simulink model "Triple_rotor_Tilerotor_model"  (R2024b)
settings: Solver=ode45  StartTime=0.0  StopTime=100  FixedStep=1e-3  RelTol=1e-3
values from neighbouring files (symbols this model uses):
  para =     [Triple_Rotors_Tilrotor_Parameters.mat]
undefined symbols (not defined in the file or in its folder): initial_height, initial_pitch, initial_vx, magnitude, rot2
libraries: simulink x9, slpidlib x5, matrix_library x4, vrlib x1
(part 2 of 3)

== system Triple_rotor_Tilerotor_model/attack_down ==
  note: 不要使用阶跃输入，会变得不幸
  Bus Creator : BusCreator  Inputs=4
  Constant : Constant  Value=Aerodynamic_switch
  Constant1 : Constant  Value=initial_theta
  Constant2 : Constant  Value=1000
  Constant3 : Constant  Value=0
  Constant4 : Constant  Value=100
  Gain : Gain  Gain=pi/180
  Gain1 : Gain  Gain=pi/180
  Ramp : simulink/Sources/Ramp  slope=slope  start=0  InitialOutput=initial_theta
  Saturation2 : Saturate  UpperLimit=inf  LowerLimit=0
  Step : Step  Commented=on  Time=0  Before=initial_theta  After=0  SampleTime=0
  Vx* : Constant  Value=100
  gamma* : Constant  Value=0
  height : Constant  Value=1000
  tag scope: Aerodynamic_switch=global, command=global, initial_Vx=global, initial_gamma=global, initial_height=global, initial_theta=global
  wires:
  Saturation2/1 -> Bus Creator/4  "theta*"
  height/1 -> Bus Creator/2  "height*"
  gamma*/1 -> Bus Creator/3  "gamma*"
  Vx*/1 -> Bus Creator/1  "Vx*"
  Bus Creator/1 -> [command]
  Constant/1 -> [Aerodynamic_switch]
  Constant1/1 -> Gain1/1
  Constant3/1 -> Gain/1
  Constant2/1 -> [initial_height]
  Constant4/1 -> [initial_Vx]
  Gain/1 -> [initial_gamma]
  Gain1/1 -> [initial_theta]
  Ramp/1 -> Saturation2/1

== system Triple_rotor_Tilerotor_model/attack_up ==
  Bus Creator : BusCreator  Inputs=4
  Constant : Constant  Value=Aerodynamic_switch
  Constant1 : Constant  Value=0
  Constant2 : Constant  Value=1000
  Constant3 : Constant  Value=0
  Constant4 : Constant  Value=100
  Step : Step  Time=0  After=final_theta  SampleTime=0
  Vx* : Constant  Value=100
  gamma* : Constant  Value=0
  height : Constant  Value=1000
  tag scope: Aerodynamic_switch=global, command=global, initial_Vx=global, initial_gamma=global, initial_height=global, initial_theta=global
  wires:
  Step/1 -> Bus Creator/4  "theta*"
  height/1 -> Bus Creator/2  "height*"
  gamma*/1 -> Bus Creator/3  "gamma*"
  Vx*/1 -> Bus Creator/1  "Vx*"
  Bus Creator/1 -> [command]
  Constant/1 -> [Aerodynamic_switch]
  Constant1/1 -> [initial_theta]
  Constant3/1 -> [initial_gamma]
  Constant2/1 -> [initial_height]
  Constant4/1 -> [initial_Vx]

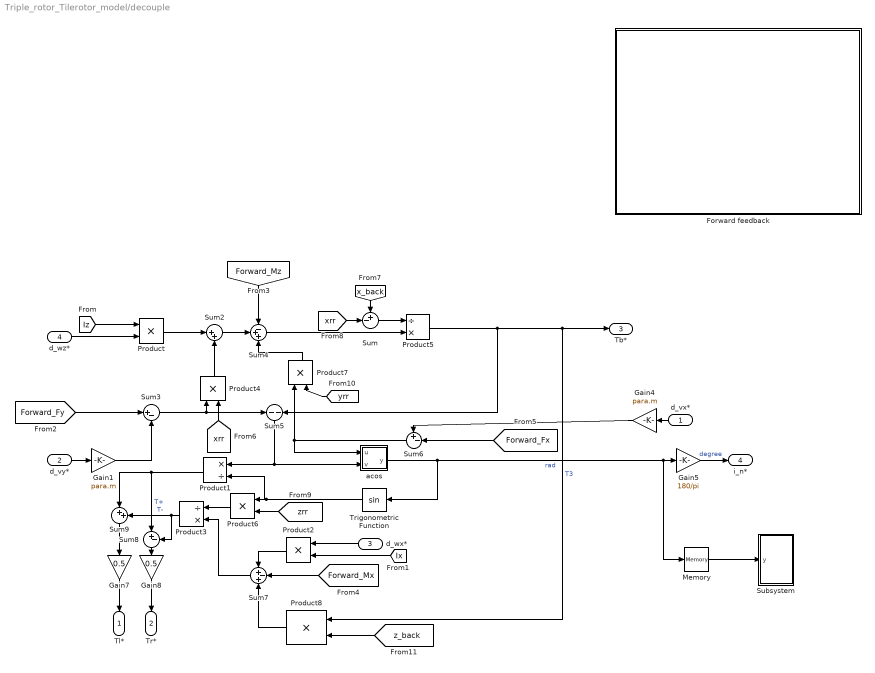
== system Triple_rotor_Tilerotor_model/decouple ==
  d_vx* : Inport
  d_vy* : Inport  Port=2
  d_wx* : Inport  Port=3
  d_wz* : Inport  Port=4
  Forward feedback : Subsystem
  Gain1 : Gain  Gain=para.m
  Gain4 : Gain  Gain=para.m
  Gain5 : Gain  Gain=180/pi
  Gain7 : Gain  Gain=0.5
  Gain8 : Gain  Gain=0.5
  Memory : Memory  InitialCondition=initial_i_n
  Product{,2,4,6..8} (6 alike) : Product
  Product1 : Product  Inputs=*/
  Product3 : Product  Inputs=/*
  Product5 : Product  Inputs=/*
  Subsystem : Subsystem
  Sum : Sum  Inputs=+-|
  Sum2 : Sum  Inputs=|++
  Sum3 : Sum  Inputs=|+-
  Sum4 : Sum  Inputs=-++
  Sum5 : Sum  Inputs=-|-
  Sum6 : Sum  Inputs=+-|
  Sum7 : Sum  Inputs=+-+
  Sum8 : Sum  Inputs=|+-
  Sum9 : Sum  Inputs=|++
  Trigonometric Function : Trigonometry
  acos : MATLAB Function  TreatAsAtomicUnit=on
  Tl* : Outport
  Tr* : Outport  Port=2
  Tb* : Outport  Port=3
  i_n* : Outport  Port=4
  wires:
  Product1/1 -> Sum8/1, Sum9/1  "T+"
  Product/1 -> Sum2/1
  [Forward_Mx] -> Sum7/2
  Gain4/1 -> Sum6/1
  Product3/1 -> Sum9/2, Sum8/2  "T-"
  [Iz] -> Product/1
  Gain1/1 -> Sum3/2
  Gain8/1 -> Tr*/1
  [Forward_Fx] -> Sum6/2
  Sum4/1 -> Product5/2
  Gain5/1 -> i_n*/1  "degree"
  [Ix] -> Product2/2
  d_vy*/1 -> Gain1/1
  Sum7/1 -> Product3/2
  d_vx*/1 -> Gain4/1
  Sum8/1 -> Gain8/1
  Sum3/1 -> Sum5/1, Product4/1
  Gain7/1 -> Tl*/1
  Product2/1 -> Sum7/1
  Trigonometric Function/1 -> Product1/2, Product6/1
  Product6/1 -> Product3/1
  d_wx*/1 -> Product2/1
  Sum9/1 -> Gain7/1
  Product4/1 -> Sum2/2
  [xrr] -> Product4/2
  [x_back] -> Sum/1
  [xrr] -> Sum/2
  Sum/1 -> Product5/1
  [zrr] -> Product6/2
  d_wz*/1 -> Product/2
  [yrr] -> Product7/2
  Product7/1 -> Sum4/3
  [z_back] -> Product8/2
  Product8/1 -> Sum7/3
  Product5/1 -> Sum5/2, Tb*/1, Product8/1  "T3"
  acos/1(y) -> Trigonometric Function/1, Memory/1, Gain5/1  "rad"
  Memory/1 -> Subsystem/1(y)
  Sum5/1 -> acos/2(v), Product1/1
  Sum6/1 -> acos/1(u), Product7/1
  [Forward_Mz] -> Sum4/1
  Sum2/1 -> Sum4/2
  [Forward_Fy] -> Sum3/1

== system Triple_rotor_Tilerotor_model/elevate2 ==
  Bus Creator : BusCreator  Inputs=4
  Constant : Constant  Value=Aerodynamic_switch
  Constant1 : Constant  Value=4
  Constant2 : Constant  Value=1000
  Constant3 : Constant  Value=0
  Constant4 : Constant  Value=100
  Constant5 : Constant  Value=-40
  Continuous Pulse Generator : DiscretePulseGenerator  PulseType=Time based  Amplitude=max_gamma  Period=200  PulseWidth=2  PhaseDelay=20
  Gain : Gain  Gain=pi/180
  Gain1 : Gain  Gain=pi/180
  Vx* : Constant  Value=100
  height : Constant  Value=1000
  theta*1 : Constant  Value=4
  tag scope: Aerodynamic_switch=global, command=global, in=global, initial_Vx=global, initial_gamma=global, initial_height=global, initial_theta=global
  wires:
  theta*1/1 -> Bus Creator/4  "theta*"
  height/1 -> Bus Creator/2  "height*"
  Continuous Pulse Generator/1 -> Bus Creator/3  "gamma*"
  Vx*/1 -> Bus Creator/1  "Vx*"
  Bus Creator/1 -> [command]
  Constant/1 -> [Aerodynamic_switch]
  Constant1/1 -> Gain1/1
  Constant3/1 -> Gain/1
  Constant2/1 -> [initial_height]
  Constant4/1 -> [initial_Vx]
  Gain/1 -> [initial_gamma]
  Gain1/1 -> [initial_theta]
  Constant5/1 -> [in]

== system Triple_rotor_Tilerotor_model/height ==
  Bus Creator : BusCreator  Inputs=4
  Constant : Constant  Value=Aerodynamic_switch
  Constant2 : Constant  Value=1000
  Constant4 : Constant  Value=100
  Constant5 : Constant  Value=0
  Constant6 : Constant  Value=0
  Gain : Gain  Gain=pi/180
  Gain1 : Gain  Gain=pi/180
  Ramp : simulink/Sources/Ramp  slope=slope  start=0  InitialOutput=1000
  Saturation2 : Saturate  UpperLimit=final_y  LowerLimit=0
  dx* : Constant  Value=100
  gamma* : Constant  Value=0
  theta* : Constant  Value=4
  tag scope: Aerodynamic_switch=global, command=global, initial_Vx=global, initial_gamma=global, initial_height=global, initial_theta=global
  wires:
  theta*/1 -> Bus Creator/4  "theta*"
  Saturation2/1 -> Bus Creator/2  "height*"
  gamma*/1 -> Bus Creator/3  "gamma*"
  Ramp/1 -> Saturation2/1
  dx*/1 -> Bus Creator/1  "Vx*"
  Bus Creator/1 -> [command]
  Constant/1 -> [Aerodynamic_switch]
  Constant2/1 -> [initial_height]
  Constant4/1 -> [initial_Vx]
  Gain1/1 -> [initial_theta]
  Constant5/1 -> Gain1/1
  Constant6/1 -> Gain/1
  Gain/1 -> [initial_gamma]

== system Triple_rotor_Tilerotor_model/observe ==
  In1 : Inport
  In2 : Inport  Port=2
  Bus Creator{1..7} (7 alike) : BusCreator  Inputs=2
  Bus Selector : BusSelector  OutputSignals=vx,vy,vz,gamma,psi,theta,wx,wy,wz
  Bus Selector1 : BusSelector  OutputSignals=vx_d,vy_d,gamma_d,theta_d
  Bus Selector2 : BusSelector  OutputSignals=wx_d,wz_d
  Demux2 : Demux  Outputs=2
  Gain5 : Gain  Gain=180/pi
  Gain6 : Gain  Gain=180/pi
  Gain7 : Gain  Gain=180/pi
  Matrix Multiply : Product  Multiplication=Matrix(*)
  Sum : Sum  Inputs=|++
  rot2(pitch) : MATLABFcn  MATLABFcn=rot2(u)  OutputDimensions=[2 2]  Output1D=off
  vx : Outport
  vy : Outport  Port=2
  <vz> : Outport  Port=3
  gamma : Outport  Port=4
  psi : Outport  Port=5
  theta : Outport  Port=6
  wx : Outport  Port=7
  <wy> : Outport  Port=8
  wz : Outport  Port=9
  i_n : Outport  Port=10
  wires:
  Bus Selector/5 -> Gain7/1  "<psi>"
  Bus Selector2/2 -> Bus Creator6/2  "<wz_d>"
  Bus Selector/7 -> Bus Creator5/1  "<wx>"
  Bus Selector/2 -> Bus Creator7/2  "<vy>"
  Bus Creator4/1 -> Gain6/1
  Bus Selector/9 -> Bus Creator6/1  "<wz>"
  Bus Creator3/1 -> Gain5/1
  Bus Selector/4 -> Bus Creator3/1  "<gamma>"
  Bus Selector1/1 -> Bus Creator1/2  "<vx_d>"
  Bus Selector/6 -> rot2(pitch)/1, Bus Creator4/1  "<theta>"
  Bus Creator7/1 -> Matrix Multiply/2
  rot2(pitch)/1 -> Matrix Multiply/1
  Demux2/2 -> Bus Creator2/1
  Gain6/1 -> theta/1  "theta"
  Bus Creator6/1 -> wz/1  "wz"
  [desire2] -> Bus Selector2/1
  Bus Selector/3 -> <vz>/1  "<vz>"
  Bus Selector1/3 -> Bus Creator3/2  "<gamma_d>"
  Bus Selector1/4 -> Bus Creator4/2  "<theta_d>"
  Bus Creator2/1 -> vy/1  "vy"
  Matrix Multiply/1 -> Demux2/1
  Bus Selector2/1 -> Bus Creator5/2  "<wx_d>"
  Demux2/1 -> Bus Creator1/1
  Bus Creator5/1 -> wx/1  "wx"
  Bus Selector1/2 -> Bus Creator2/2  "<vy_d>"
  [desire] -> Bus Selector1/1
  Bus Selector/8 -> <wy>/1  "<wy>"
  Bus Selector/1 -> Bus Creator7/1  "<vx>"
  In1/1 -> Bus Selector/1
  Gain7/1 -> psi/1  "psi"
  Gain5/1 -> gamma/1  "gamma"
  Bus Creator1/1 -> vx/1  "vx"
  Sum/1 -> i_n/1
  In2/1 -> Sum/1
  [in] -> Sum/2

== system Triple_rotor_Tilerotor_model/rotation_speed ==
  Tl_in : Inport
  Tr_in : Inport  Port=2
  Tb_in : Inport  Port=3
  i_n_in : Inport  Port=4
  Bus Creator : BusCreator  Inputs=2
  Demux : Demux  Outputs=2
  Gain : Gain  Gain=2/para.CT/para.rho/power(para.R,4)
  Gain1 : Gain  Gain=2/para.CT/para.rho/power(para.R,4)
  Saturation1 : Saturate  UpperLimit=maxrot  LowerLimit=minrot
  Saturation2 : Saturate  UpperLimit=inf  LowerLimit=1
  Saturation3 : Saturate  UpperLimit=maxi_n  LowerLimit=mini_n
  Saturation4 : Saturate  UpperLimit=maxrot  LowerLimit=minrot
  Saturation5 : Saturate  UpperLimit=para.maxrot  LowerLimit=minrot
  Scope : Scope  NumInputPorts=3
  Signed Square Root : Sqrt  Operator=signedSqrt
  Sqrt : Sqrt  OutputSignalType=real
  wl : Outport
  wr : Outport  Port=2
  wb : Outport  Port=3
  i_n : Outport  Port=4
  wires:
  Tl_in/1 -> Bus Creator/1  "T1"
  Sqrt/1 -> Demux/1
  Tb_in/1 -> Gain1/1  "T3"
  Tr_in/1 -> Bus Creator/2  "T2"
  Demux/2 -> Scope/2, Saturation4/1
  Bus Creator/1 -> Saturation2/1
  Signed Square Root/1 -> Scope/3, Saturation5/1
  Demux/1 -> Saturation1/1, Scope/1
  i_n_in/1 -> Saturation3/1
  Saturation3/1 -> i_n/1  "T3"
  Saturation1/1 -> wl/1  "T1"
  Saturation5/1 -> wb/1  "T1"
  Saturation2/1 -> Gain/1
  Saturation4/1 -> wr/1  "T1"
  Gain/1 -> Sqrt/1
  Gain1/1 -> Signed Square Root/1

== system Triple_rotor_Tilerotor_model/slowdown ==
  Bus Creator : BusCreator  Inputs=4
  Constant : Constant  Value=Aerodynamic_switch
  Constant1 : Constant  Value=0
  Constant2 : Constant  Value=1000
  Constant3 : Constant  Value=0
  Constant4 : Constant  Value=initial_velocity
  Ramp : simulink/Sources/Ramp  slope=-(initial_velocity)/10  start=0  InitialOutput=initial_velocity
  Saturation2 : Saturate  UpperLimit=inf  LowerLimit=0
  gamma* : Constant  Value=0
  height : Constant  Value=1000
  theta* : Constant  Value=0
  tag scope: Aerodynamic_switch=global, command=global, initial_Vx=global, initial_gamma=global, initial_height=global, initial_theta=global
  wires:
  theta*/1 -> Bus Creator/4  "theta*"
  height/1 -> Bus Creator/2  "height*"
  gamma*/1 -> Bus Creator/3  "gamma*"
  Saturation2/1 -> Bus Creator/1  "Vx*"
  Bus Creator/1 -> [command]
  Constant/1 -> [Aerodynamic_switch]
  Constant1/1 -> [initial_theta]
  Constant3/1 -> [initial_gamma]
  Constant2/1 -> [initial_height]
  Constant4/1 -> [initial_Vx]
  Ramp/1 -> Saturation2/1

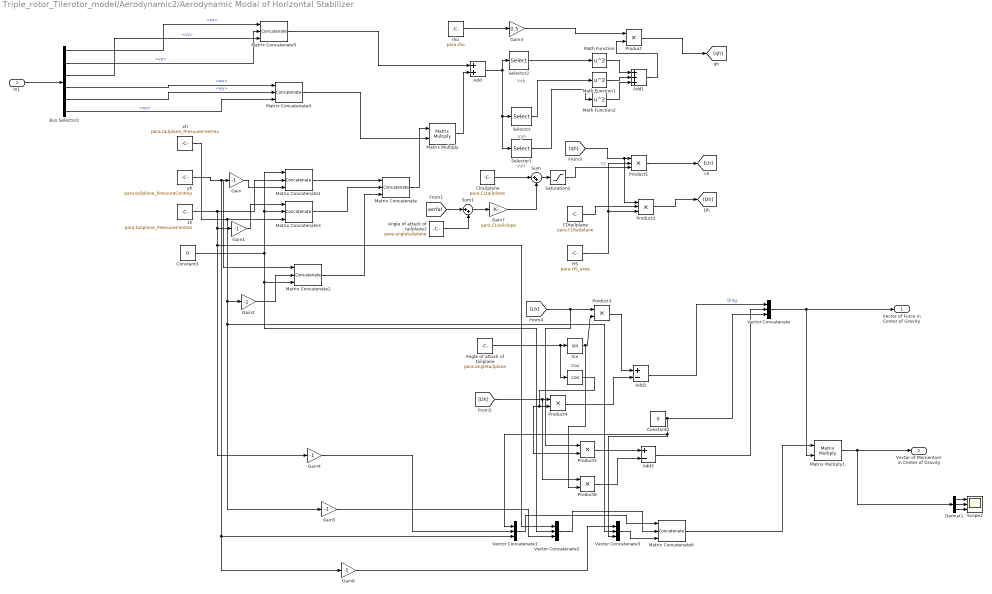
== system Triple_rotor_Tilerotor_model/Aerodynamic2/Aerodynamic Modal of Horizontal Stabilizer ==
  note: Vzh
  note: Vyh
  note: Vxh
  In1 : Inport
  Add : Sum
  Add1 : Sum  Inputs=+++
  Add2 : Sum  Inputs=+-
  Add3 : Sum  Inputs=+-
  Angle of attack of tailplane : Constant  Value=para.angletailplane
  Angle of attack of tailplane1 : Constant  Value=para.angletailplane
  Bus Selector2 : BusSelector  OutputSignals=vx,vy,vz,wx,wy,wz
  CDtailplane : Constant  Value=para.CDtailplane
  Cltailplane : Constant  Value=para.CLtailplane
  Constant3 : Constant  Value=0
  Constant4 : Constant  Value=0
  Cos : Trigonometry  Operator=cos
  Demux1 : Demux  Outputs=3
  Gain{,1..2,4..6} (6 alike) : Gain  Gain=-1
  Gain3 : Gain  Gain=0.5
  Gain7 : Gain  Gain=para.CLtailslope
  HS : Constant  Value=para.HS_area
  Math Function : Math  Operator=square
  Math Function1 : Math  Operator=square
  Math Function2 : Math  Operator=square
  Matrix Concatenate : Concatenate  NumInputs=3  Mode=Multidimensional array  ConcatenateDimension=2
  Matrix Concatenate{1..5} (5 alike) : Concatenate  NumInputs=3  ConcatenateDimension=2
  Matrix Concatenate6 : Concatenate  NumInputs=3  Mode=Multidimensional array  ConcatenateDimension=2
  Matrix Multiply : Product  Multiplication=Matrix(*)
  Matrix Multiply1 : Product  Multiplication=Matrix(*)
  Product{,3..6} (5 alike) : Product
  Product1 : Product  Inputs=3
  Product2 : Product  Inputs=3
  Saturation2 : Saturate  UpperLimit=1  LowerLimit=-1
  Scope2 : Scope  NumInputPorts=3
  Selector : Selector  InputPortWidth=3  IndexOptions=Index vector (dialog)  Indices=2  OutputSizes=1
  Selector1 : Selector  InputPortWidth=3  IndexOptions=Index vector (dialog)  Indices=3  OutputSizes=1
  Selector2 : Selector  InputPortWidth=3  IndexOptions=Index vector (dialog)  Indices=[1]  OutputSizes=1
  Sin : Trigonometry
  Sum : Sum  Inputs=|++
  Sum1 : Sum  Inputs=|++
  Vector Concatenate{,1..3} (4 alike) : Concatenate  NumInputs=3
  rho : Constant  Value=para.rho
  xh : Constant  Value=para.tailplane_PressureCentrex
  yh : Constant  Value=para.tailplane_PressureCentrey
  zh : Constant  Value=para.tailplane_PressureCentrez
  Vector of Force in Center of Gravity : Outport
  Vector of Momentum in Center of Gravity : Outport  Port=2
  wires:
  CDtailplane/1 -> Product2/2
  rho/1 -> Gain3/1
  Matrix Concatenate6/1 -> Matrix Multiply1/1
  zh/1 -> Vector Concatenate2/1, Gain4/1, Gain1/1, Matrix Concatenate1/2
  Matrix Concatenate4/1 -> Matrix Multiply/2
  Matrix Concatenate3/1 -> Matrix Concatenate/2
  Add1/1 -> Product/2
  [qh] -> Product2/1, Product1/1
  yh/1 -> Vector Concatenate1/3, Gain6/1, Matrix Concatenate2/1, Gain/1
  Sin/1 -> Product6/2, Product3/2
  Product2/1 -> [Dh]
  Vector Concatenate2/1 -> Matrix Concatenate6/2
  Add/1 -> Selector1/1, Selector/1, Selector2/1
  Vector Concatenate1/1 -> Matrix Concatenate6/1
  Sum/1 -> Saturation2/1
  Matrix Concatenate2/1 -> Matrix Concatenate/3
  Gain4/1 -> Vector Concatenate1/2
  xh/1 -> Vector Concatenate3/2, Gain5/1, Gain2/1, Matrix Concatenate3/3
  Bus Selector2/3 -> Matrix Concatenate5/3  "<vz>"
  Math Function/1 -> Add1/1
  HS/1 -> Product2/3, Product1/2
  Bus Selector2/1 -> Matrix Concatenate5/1  "<vx>"
  [Dh] -> Product4/1, Product6/1
  Selector1/1 -> Math Function2/1
  [Lh] -> Product5/1, Product3/1
  Math Function1/1 -> Add1/2
  Constant3/1 -> Matrix Concatenate2/3, Vector Concatenate2/2, Matrix Concatenate3/2, Matrix Concatenate1/1
  Gain3/1 -> Product/1
  In1/1 -> Bus Selector2/1
  Angle of attack of tailplane/1 -> Cos/1, Sin/1
  Add3/1 -> Vector Concatenate/2
  Gain6/1 -> Vector Concatenate3/1
  Product/1 -> [qh]
  Selector/1 -> Math Function1/1
  Gain5/1 -> Vector Concatenate2/3
  Bus Selector2/5 -> Matrix Concatenate4/2  "<wy>"
  Constant4/1 -> Vector Concatenate3/3, Vector Concatenate1/1, Vector Concatenate/3
  Gain2/1 -> Matrix Concatenate2/2
  Bus Selector2/2 -> Matrix Concatenate5/2  "<vy>"
  Matrix Multiply/1 -> Add/2
  Vector Concatenate/1 -> Vector of Force in Center of Gravity/1, Matrix Multiply1/2
  Product3/1 -> Add2/1
  Bus Selector2/4 -> Matrix Concatenate4/1  "<wx>"
  Product4/1 -> Add2/2
  Bus Selector2/6 -> Matrix Concatenate4/3  "<wz>"
  Product6/1 -> Add3/2
  Gain/1 -> Matrix Concatenate1/3
  Matrix Concatenate1/1 -> Matrix Concatenate/1
  Cos/1 -> Product4/2, Product5/2
  Gain1/1 -> Matrix Concatenate3/1
  Matrix Concatenate5/1 -> Add/1
  Matrix Concatenate/1 -> Matrix Multiply/1
  Vector Concatenate3/1 -> Matrix Concatenate6/3
  Selector2/1 -> Math Function/1
  Math Function2/1 -> Add1/3
  Product5/1 -> Add3/1
  Product1/1 -> [Lh]
  Cltailplane/1 -> Sum/1
  Gain7/1 -> Sum/2
  Sum1/1 -> Gain7/1
  [aerfaf] -> Sum1/1
  Angle of attack of tailplane1/1 -> Sum1/2
  Saturation2/1 -> Product1/3  "T3"
  Add2/1 -> Vector Concatenate/1  "Drag"
  Demux1/3 -> Scope2/3
  Demux1/1 -> Scope2/1
  Matrix Multiply1/1 -> Demux1/1, Vector of Momentum in Center of Gravity/1
  Demux1/2 -> Scope2/2

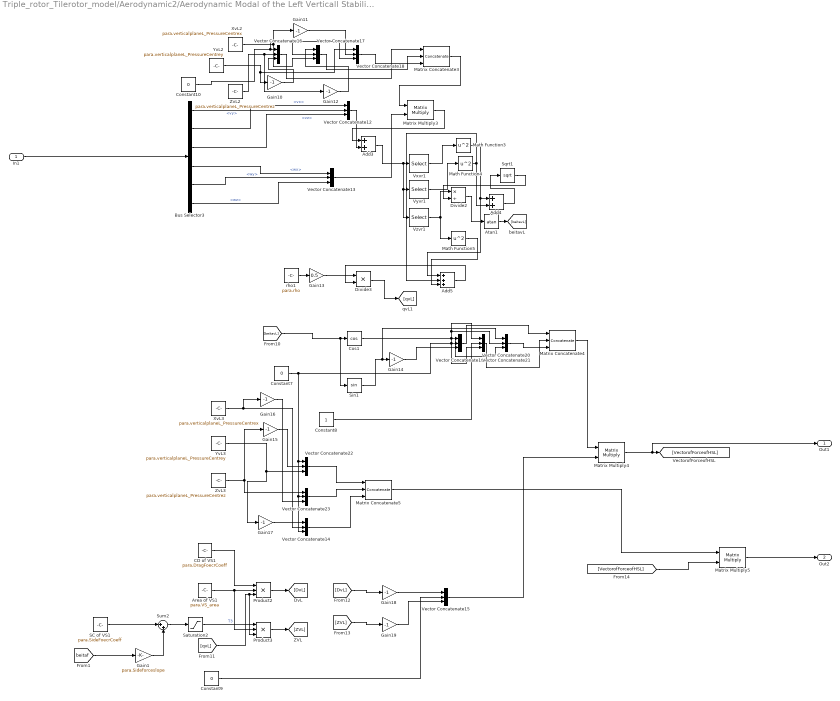
== system Triple_rotor_Tilerotor_model/Aerodynamic2/Aerodynamic Modal of the Left Verticall Stabilizer ==
  In1 : Inport
  Add3 : Sum
  Add4 : Sum
  Add5 : Sum  Inputs=+++
  Area of VS1 : Constant  Value=para.VS_area
  Atan1 : Trigonometry  Operator=atan
  Bus Selector3 : BusSelector  OutputSignals=vy,vx,vz,wx,wy,wz
  CD of VS1 : Constant  Value=para.DragFoecrCoeff
  Constant10 : Constant  Value=0
  Constant7 : Constant  Value=0
  Constant8 : Constant
  Constant9 : Constant  Value=0
  Cos1 : Trigonometry  Operator=cos
  Divide2 : Product  Inputs=*/
  Divide3 : Product  Inputs=**
  Gain1 : Gain  Gain=para.Sideforceslope
  Gain{10..12,14..19} (9 alike) : Gain  Gain=-1
  Gain13 : Gain  Gain=0.5
  Math Function3 : Math  Operator=square
  Math Function4 : Math  Operator=square
  Math Function5 : Math  Operator=square
  Matrix Concatenate3 : Concatenate  NumInputs=3  Mode=Multidimensional array  ConcatenateDimension=2
  Matrix Concatenate4 : Concatenate  NumInputs=3  Mode=Multidimensional array  ConcatenateDimension=2
  Matrix Concatenate5 : Concatenate  NumInputs=3  Mode=Multidimensional array  ConcatenateDimension=2
  Matrix Multiply3 : Product  Multiplication=Matrix(*)
  Matrix Multiply4 : Product  Multiplication=Matrix(*)
  Matrix Multiply5 : Product  Multiplication=Matrix(*)
  Product2 : Product  Inputs=3
  Product3 : Product  Inputs=3
  SC of VS1 : Constant  Value=para.SideFoecrCoeff
  Saturation2 : Saturate  UpperLimit=1  LowerLimit=-1
  Sin1 : Trigonometry
  Sqrt1 : Sqrt
  Sum2 : Sum  Inputs=|++
  Vector Concatenate{12..23} (12 alike) : Concatenate  NumInputs=3
  Vxvr1 : Selector  InputPortWidth=3  IndexOptions=Index vector (dialog)  Indices=[1]  OutputSizes=1
  Vyvr1 : Selector  InputPortWidth=3  IndexOptions=Index vector (dialog)  Indices=[2]  OutputSizes=1
  Vzvr1 : Selector  InputPortWidth=3  IndexOptions=Index vector (dialog)  Indices=[3]  OutputSizes=1
  XvL2 : Constant  Value=para.verticalplaneL_PressureCentrex
  XvL3 : Constant  Value=para.verticalplaneL_PressureCentrex
  YvL2 : Constant  Value=para.verticalplaneL_PressureCentrey
  YvL3 : Constant  Value=para.verticalplaneL_PressureCentrey
  ZvL2 : Constant  Value=para.verticalplaneL_PressureCentrez
  ZvL3 : Constant  Value=para.verticalplaneL_PressureCentrez
  rho1 : Constant  Value=para.rho
  Out1 : Outport
  Out2 : Outport  Port=2
  wires:
  Vyvr1/1 -> Math Function4/1
  Constant7/1 -> Vector Concatenate14/3, Vector Concatenate23/2, Vector Concatenate22/1, Vector Concatenate20/1, Vector Concatenate21/2, Vector Concatenate19/2, Vector Concatenate20/3
  Bus Selector3/5 -> Vector Concatenate13/2  "<wy>"
  Bus Selector3/3 -> Vector Concatenate12/3  "<vz>"
  Matrix Multiply4/1 -> Out1/1, [VectorofForceofHSL]
  Sum2/1 -> Saturation2/1
  Gain19/1 -> Vector Concatenate15/3
  Constant9/1 -> Vector Concatenate15/2
  Add3/1 -> Vyvr1/1, Vzvr1/1, Vxvr1/1
  Matrix Multiply3/1 -> Add3/1
  XvL3/1 -> Vector Concatenate14/2, Gain16/1
  Divide3/1 -> [qvL]
  Math Function4/1 -> Add4/2, Add5/2
  Constant8/1 -> Vector Concatenate20/2
  [DvL] -> Gain18/1
  [VectorofForceofHSL] -> Matrix Multiply5/2
  [ZVL] -> Gain19/1
  Gain10/1 -> Vector Concatenate16/3
  Vector Concatenate22/1 -> Matrix Concatenate5/1
  Gain12/1 -> Vector Concatenate17/1
  Vector Concatenate21/1 -> Matrix Concatenate4/3
  Constant10/1 -> Vector Concatenate17/2, Vector Concatenate18/3, Vector Concatenate16/1
  YvL2/1 -> Vector Concatenate18/1, Gain10/1
  Bus Selector3/6 -> Vector Concatenate13/3  "<wz>"
  Gain13/1 -> Divide3/1
  Gain18/1 -> Vector Concatenate15/1
  Bus Selector3/4 -> Vector Concatenate13/1  "<wx>"
  Cos1/1 -> Vector Concatenate21/3, Vector Concatenate19/1
  Gain16/1 -> Vector Concatenate23/3
  Matrix Concatenate4/1 -> Matrix Multiply4/1
  Bus Selector3/1 -> Vector Concatenate12/2  "<vy>"
  Math Function5/1 -> Add5/3
  Vector Concatenate23/1 -> Matrix Concatenate5/2
  YvL3/1 -> Gain17/1, Vector Concatenate22/3
  Math Function3/1 -> Add5/1, Add4/1
  Add4/1 -> Sqrt1/1
  Atan1/1 -> [beitavL]
  Vxvr1/1 -> Math Function3/1
  Product3/1 -> [ZVL]
  Sin1/1 -> Vector Concatenate21/1, Gain14/1
  Sqrt1/1 -> Divide2/2
  [beitavL] -> Sin1/1, Cos1/1
  Vector Concatenate13/1 -> Matrix Multiply3/2
  Matrix Concatenate3/1 -> Matrix Multiply3/1
  Area of VS1/1 -> Product3/2, Product2/2
  Vzvr1/1 -> Math Function5/1, Divide2/1
  Vector Concatenate12/1 -> Add3/2
  Vector Concatenate18/1 -> Matrix Concatenate3/3
  Product2/1 -> [DvL]
  rho1/1 -> Gain13/1
  Gain11/1 -> Vector Concatenate18/2
  Gain14/1 -> Vector Concatenate19/3
  Vector Concatenate20/1 -> Matrix Concatenate4/2
  Vector Concatenate14/1 -> Matrix Concatenate5/3
  Vector Concatenate17/1 -> Matrix Concatenate3/2
  ZvL2/1 -> Vector Concatenate16/2, Gain12/1
  Bus Selector3/2 -> Vector Concatenate12/1  "<vx>"
  XvL2/1 -> Gain11/1, Vector Concatenate17/3
  Vector Concatenate16/1 -> Matrix Concatenate3/1
  [qvL] -> Product3/3, Product2/3
  Divide2/1 -> Atan1/1
  Vector Concatenate19/1 -> Matrix Concatenate4/1
  CD of VS1/1 -> Product2/1
  Gain17/1 -> Vector Concatenate14/1
  Matrix Concatenate5/1 -> Matrix Multiply5/1
  Add5/1 -> Divide3/2
  In1/1 -> Bus Selector3/1
  ZvL3/1 -> Vector Concatenate23/1, Gain15/1
  Gain15/1 -> Vector Concatenate22/2
  SC of VS1/1 -> Sum2/1
  Gain1/1 -> Sum2/2
  [beitaf] -> Gain1/1
  Saturation2/1 -> Product3/1  "T3"
  Vector Concatenate15/1 -> Matrix Multiply4/2
  Matrix Multiply5/1 -> Out2/1

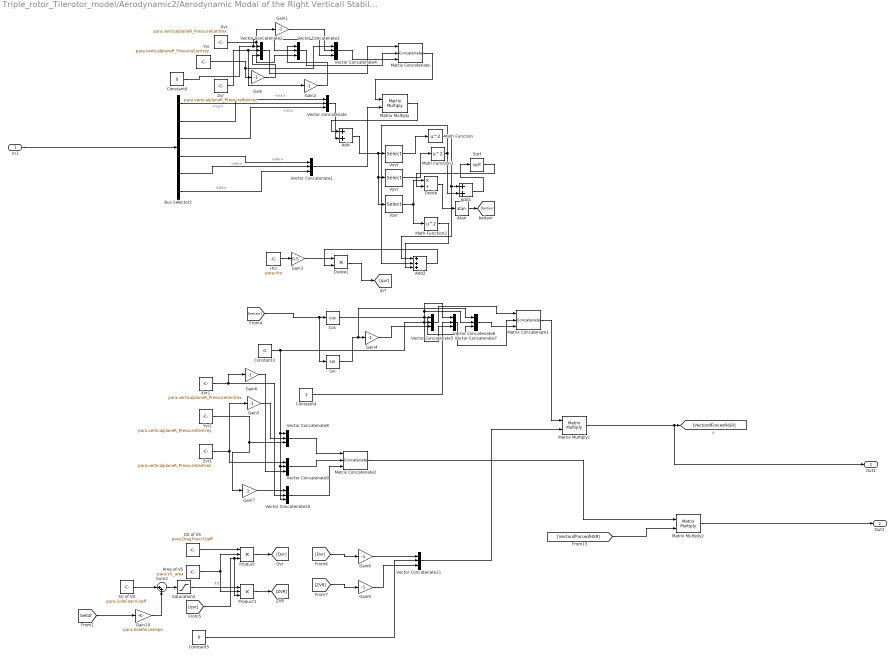
== system Triple_rotor_Tilerotor_model/Aerodynamic2/Aerodynamic Modal of the Right Verticall Stabilizer ==
  In1 : Inport
  Add : Sum
  Add1 : Sum
  Add2 : Sum  Inputs=+++
  Area of VS : Constant  Value=para.VS_area
  Atan : Trigonometry  Operator=atan
  Bus Selector2 : BusSelector  OutputSignals=vy,vx,vz,wx,wy,wz
  CD of VS : Constant  Value=para.DragFoecrCoeff
  Constant3 : Constant  Value=0
  Constant4 : Constant
  Constant5 : Constant  Value=0
  Constant6 : Constant  Value=0
  Cos : Trigonometry  Operator=cos
  Divide : Product  Inputs=*/
  Divide1 : Product  Inputs=**
  Gain{,1..2,4..9} (9 alike) : Gain  Gain=-1
  Gain10 : Gain  Gain=para.Sideforceslope
  Gain3 : Gain  Gain=0.5
  Math Function : Math  Operator=square
  Math Function1 : Math  Operator=square
  Math Function2 : Math  Operator=square
  Matrix Concatenate : Concatenate  NumInputs=3  Mode=Multidimensional array  ConcatenateDimension=2
  Matrix Concatenate1 : Concatenate  NumInputs=3  Mode=Multidimensional array  ConcatenateDimension=2
  Matrix Concatenate2 : Concatenate  NumInputs=3  Mode=Multidimensional array  ConcatenateDimension=2
  Matrix Multiply : Product  Multiplication=Matrix(*)
  Matrix Multiply1 : Product  Multiplication=Matrix(*)
  Matrix Multiply2 : Product  Multiplication=Matrix(*)
  Product : Product  Inputs=3
  Product1 : Product  Inputs=3
  SC of VS : Constant  Value=para.SideFoecrCoeff
  Saturation2 : Saturate  UpperLimit=1  LowerLimit=-1
  Sin : Trigonometry
  Sqrt : Sqrt
  Sum2 : Sum  Inputs=|++
  Vector Concatenate{,1..11} (12 alike) : Concatenate  NumInputs=3
  Vxvr : Selector  InputPortWidth=3  IndexOptions=Index vector (dialog)  Indices=[1]  OutputSizes=1
  Vyvr : Selector  InputPortWidth=3  IndexOptions=Index vector (dialog)  Indices=[2]  OutputSizes=1
  Vzvr : Selector  InputPortWidth=3  IndexOptions=Index vector (dialog)  Indices=[3]  OutputSizes=1
  Xvr : Constant  Value=para.verticalplaneR_PressureCentrex
  Xvr1 : Constant  Value=para.verticalplaneR_PressureCentrex
  Yvr : Constant  Value=para.verticalplaneR_PressureCentrey
  Yvr1 : Constant  Value=para.verticalplaneR_PressureCentrey
  Zvr : Constant  Value=para.verticalplaneR_PressureCentrez
  Zvr1 : Constant  Value=para.verticalplaneR_PressureCentrez
  rho : Constant  Value=para.rho
  Out1 : Outport
  Out2 : Outport  Port=2
  wires:
  Zvr/1 -> Vector Concatenate2/2, Gain2/1
  Sin/1 -> Vector Concatenate7/1, Gain4/1
  Divide1/1 -> [qvr]
  Matrix Multiply1/1 -> Out1/1, [VectorofForceofHSR]
  Vector Concatenate11/1 -> Matrix Multiply1/2
  [beitavr] -> Sin/1, Cos/1
  Constant6/1 -> Vector Concatenate3/2, Vector Concatenate4/3, Vector Concatenate2/1
  Xvr/1 -> Gain1/1, Vector Concatenate3/3
  Bus Selector2/5 -> Vector Concatenate1/2  "<wy>"
  Gain8/1 -> Vector Concatenate11/1
  Cos/1 -> Vector Concatenate7/3, Vector Concatenate5/1
  CD of VS/1 -> Product/1
  Matrix Concatenate2/1 -> Matrix Multiply2/1
  Gain7/1 -> Vector Concatenate10/1
  Vector Concatenate1/1 -> Matrix Multiply/2
  Area of VS/1 -> Product1/2, Product/2
  Vector Concatenate5/1 -> Matrix Concatenate1/1
  [qvr] -> Product1/3, Product/3
  Matrix Concatenate1/1 -> Matrix Multiply1/1
  Bus Selector2/2 -> Vector Concatenate/1  "<vx>"
  [ZVR] -> Gain9/1
  Vector Concatenate4/1 -> Matrix Concatenate/3
  Vxvr/1 -> Math Function/1
  Math Function1/1 -> Add1/2, Add2/2
  Matrix Multiply/1 -> Add/1
  Add1/1 -> Sqrt/1
  Vector Concatenate10/1 -> Matrix Concatenate2/3
  Math Function2/1 -> Add2/3
  Vector Concatenate2/1 -> Matrix Concatenate/1
  Xvr1/1 -> Vector Concatenate10/2, Gain6/1
  Bus Selector2/4 -> Vector Concatenate1/1  "<wx>"
  [VectorofForceofHSR] -> Matrix Multiply2/2
  Gain1/1 -> Vector Concatenate4/2
  Product/1 -> [Dvr]
  Atan/1 -> [beitavr]
  Vector Concatenate3/1 -> Matrix Concatenate/2
  Gain6/1 -> Vector Concatenate9/3
  Gain/1 -> Vector Concatenate2/3
  Add/1 -> Vyvr/1, Vzvr/1, Vxvr/1
  Vector Concatenate6/1 -> Matrix Concatenate1/2
  rho/1 -> Gain3/1
  Gain2/1 -> Vector Concatenate3/1
  Gain4/1 -> Vector Concatenate5/3
  Yvr/1 -> Vector Concatenate4/1, Gain/1
  Vector Concatenate/1 -> Add/2
  Vector Concatenate7/1 -> Matrix Concatenate1/3
  Gain9/1 -> Vector Concatenate11/3
  Sum2/1 -> Saturation2/1
  Matrix Concatenate/1 -> Matrix Multiply/1
  Vzvr/1 -> Math Function2/1, Divide/1
  Bus Selector2/3 -> Vector Concatenate/3  "<vz>"
  Yvr1/1 -> Gain7/1, Vector Concatenate8/3
  Product1/1 -> [ZVR]
  Bus Selector2/6 -> Vector Concatenate1/3  "<wz>"
  Math Function/1 -> Add2/1, Add1/1
  Zvr1/1 -> Vector Concatenate9/1, Gain5/1
  Sqrt/1 -> Divide/2
  Vector Concatenate9/1 -> Matrix Concatenate2/2
  Constant3/1 -> Vector Concatenate10/3, Vector Concatenate9/2, Vector Concatenate8/1, Vector Concatenate6/1, Vector Concatenate7/2, Vector Concatenate5/2, Vector Concatenate6/3
  Vyvr/1 -> Math Function1/1
  Vector Concatenate8/1 -> Matrix Concatenate2/1
  Constant5/1 -> Vector Concatenate11/2
  Gain3/1 -> Divide1/1
  Constant4/1 -> Vector Concatenate6/2
  Bus Selector2/1 -> Vector Concatenate/2  "<vy>"
  Add2/1 -> Divide1/2
  Divide/1 -> Atan/1
  Gain5/1 -> Vector Concatenate8/2
  In1/1 -> Bus Selector2/1
  [beitaf] -> Gain10/1
  SC of VS/1 -> Sum2/1
  Gain10/1 -> Sum2/2
  Saturation2/1 -> Product1/1  "T3"
  [Dvr] -> Gain8/1
  Matrix Multiply2/1 -> Out2/1

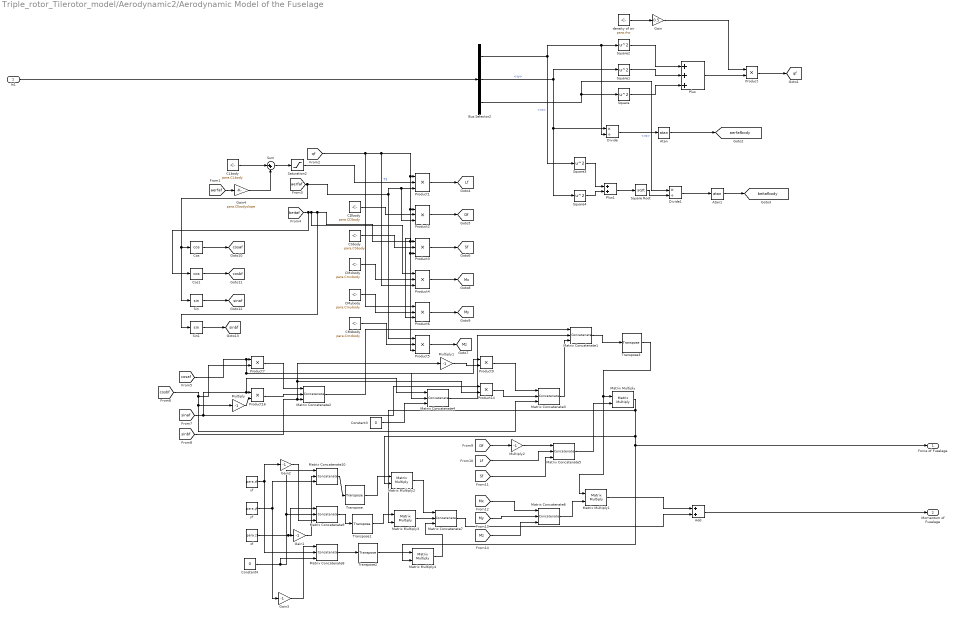
== system Triple_rotor_Tilerotor_model/Aerodynamic2/Aerodynamic Model of the Fuselage ==
  In1 : Inport
  Add : Sum
  Atan : Trigonometry  Operator=atan
  Atan1 : Trigonometry  Operator=atan
  Bus Selector2 : BusSelector  OutputSignals=vx,vy,vz
  CDbody : Constant  Value=para.CDbody
  CLbody : Constant  Value=para.CLbody
  CMxbody : Constant  Value=para.Cmxbody
  CMybody : Constant  Value=para.Cmybody
  CMzbody : Constant  Value=para.Cmzbody
  CSbody : Constant  Value=para.CSbody
  Constant3 : Constant  Value=0
  Constant4 : Constant  Value=0
  Cos : Trigonometry  Operator=cos
  Cos1 : Trigonometry  Operator=cos
  Divide : Product  Inputs=*/
  Divide1 : Product  Inputs=*/
  Gain : Gain  Gain=0.5
  Gain1 : Gain  Gain=-1
  Gain2 : Gain  Gain=-1
  Gain3 : Gain  Gain=-1
  Gain4 : Gain  Gain=para.Clbodyslope
  Matrix Concatenate1 : Concatenate  NumInputs=3  Mode=Multidimensional array  ConcatenateDimension=2
  Matrix Concatenate{2..10} (9 alike) : Concatenate  NumInputs=3  ConcatenateDimension=2
  Matrix Multiply{,1..4} (5 alike) : Product  Multiplication=Matrix(*)
  Multiply : Gain  Gain=-1
  Multiply1 : Gain  Gain=-1
  Multiply2 : Gain  Gain=-1
  Plus : Sum  Inputs=+++
  Plus1 : Sum
  Product{,7,9,14,16} (5 alike) : Product
  Product{1..6} (6 alike) : Product  Inputs=3
  Saturation2 : Saturate  UpperLimit=3  LowerLimit=-1
  Sin : Trigonometry
  Sin1 : Trigonometry
  Square{,1..4} (5 alike) : Math  Operator=square
  Square Root : Sqrt
  Sum : Sum  Inputs=|++
  Transpose{,1..3} (4 alike) : matrix_library/Transpose
  density of air : Constant  Value=para.rho
  xf : Constant  Value=para.xf
  yf : Constant  Value=para.yf
  zf : Constant  Value=para.zf
  Force of Fuselage : Outport
  Momentum of Fuselage : Outport  Port=2
  tag scope: Df=global, Lf=global, Mx=global, My=global, Mz=global, Sf=global, aerfafbody=global, beitafbody=global, cosaf=global, cosbf=global, qf=global, sinaf=global, sinbf=global
  wires:
  Matrix Concatenate8/1 -> Transpose2/1
  [cosbf] -> Multiply/1, Matrix Concatenate3/3, Product7/2
  CDbody/1 -> Product2/2
  Square1/1 -> Plus/2
  Product5/1 -> [Mz]
  Multiply/1 -> Product16/2
  Multiply1/1 -> Product9/2
  CMxbody/1 -> Product4/2
  Atan1/1 -> [beitafbody]
  Sum/1 -> Saturation2/1
  Bus Selector2/3 -> Divide1/1, Square/1  "<vz>"
  Constant4/1 -> Matrix Concatenate8/3, Matrix Concatenate9/2, Matrix Concatenate10/1
  Gain2/1 -> Matrix Concatenate9/3
  Matrix Multiply1/1 -> Add/1
  In1/1 -> Bus Selector2/1
  Matrix Concatenate2/1 -> Matrix Concatenate1/1
  [aerfaf] -> Sin/1, Cos/1, Product5/1, Product1/3, Product2/3
  Matrix Multiply4/1 -> Matrix Concatenate7/3
  density of air/1 -> Gain/1
  xf/1 -> Matrix Concatenate8/2, Gain2/1
  yf/1 -> Gain3/1, Matrix Concatenate10/3
  [qf] -> Product6/1, Product4/3, Product5/3, Product3/3, Product2/1, Product1/1
  [Mx] -> Matrix Concatenate6/1
  Product9/1 -> Matrix Concatenate3/1
  [beitaf] -> Cos1/1, Product4/1, Sin1/1, Product6/3, Product3/1
  [Sf] -> Matrix Concatenate5/3
  Square2/1 -> Plus/1
  Square Root/1 -> Divide1/2
  Matrix Concatenate6/1 -> Matrix Multiply1/2
  Gain/1 -> Product/1
  CMzbody/1 -> Product5/2
  Divide1/1 -> Atan1/1
  Cos1/1 -> [cosbf]
  [sinaf] -> Product14/1, Matrix Concatenate4/1, Product16/1
  Transpose1/1 -> Matrix Multiply3/1
  [sinbf] -> Multiply1/1, Product14/2, Matrix Concatenate2/3
  Cos/1 -> [cosaf]
  Matrix Concatenate5/1 -> Matrix Multiply/2
  Bus Selector2/2 -> Square1/1, Divide/1, Square4/1  "<vy>"
  Matrix Multiply2/1 -> Matrix Concatenate7/1
  CSbody/1 -> Product3/2
  Multiply2/1 -> Matrix Concatenate5/1
  Transpose2/1 -> Matrix Multiply4/1
  Bus Selector2/1 -> Square3/1, Square2/1, Divide/2  "<vx>"
  CMybody/1 -> Product6/2
  Square/1 -> Plus/3
  Sin/1 -> [sinaf]
  Product3/1 -> [Sf]
  Transpose/1 -> Matrix Multiply2/1
  Atan/1 -> [aerfafbody]
  Matrix Concatenate7/1 -> Add/2
  Product/1 -> [qf]
  Matrix Concatenate4/1 -> Matrix Concatenate1/2
  [cosaf] -> Matrix Concatenate4/2, Product9/1, Product7/1
  Matrix Concatenate1/1 -> Transpose3/1
  Product14/1 -> Matrix Concatenate3/2
  zf/1 -> Matrix Concatenate9/1, Gain1/1
  Matrix Concatenate3/1 -> Matrix Concatenate1/3
  Matrix Concatenate9/1 -> Transpose1/1
  Square4/1 -> Plus1/2
  [Df] -> Multiply2/1
  [Lf] -> Matrix Concatenate5/2
  Plus1/1 -> Square Root/1
  Product2/1 -> [Df]
  Product4/1 -> [Mx]
  Product1/1 -> [Lf]
  Square3/1 -> Plus1/1
  Product6/1 -> [My]
  Sin1/1 -> [sinbf]
  Product16/1 -> Matrix Concatenate2/2
  Plus/1 -> Product/2
  Divide/1 -> Atan/1
  [Mz] -> Matrix Concatenate6/3
  Product7/1 -> Matrix Concatenate2/1
  Constant3/1 -> Matrix Concatenate4/3
  Gain3/1 -> Matrix Concatenate8/1
  Gain1/1 -> Matrix Concatenate10/2
  Matrix Concatenate10/1 -> Transpose/1
  Matrix Multiply3/1 -> Matrix Concatenate7/2
  [My] -> Matrix Concatenate6/2
  Transpose3/1 -> Matrix Multiply1/1, Matrix Multiply/1
  Gain4/1 -> Sum/2
  [aerfaf] -> Gain4/1
  CLbody/1 -> Sum/1
  Saturation2/1 -> Product1/2  "T3"
  Matrix Multiply/1 -> Matrix Multiply4/2, Force of Fuselage/1, Matrix Multiply2/2, Matrix Multiply3/2
  Add/1 -> Momentum of Fuselage/1

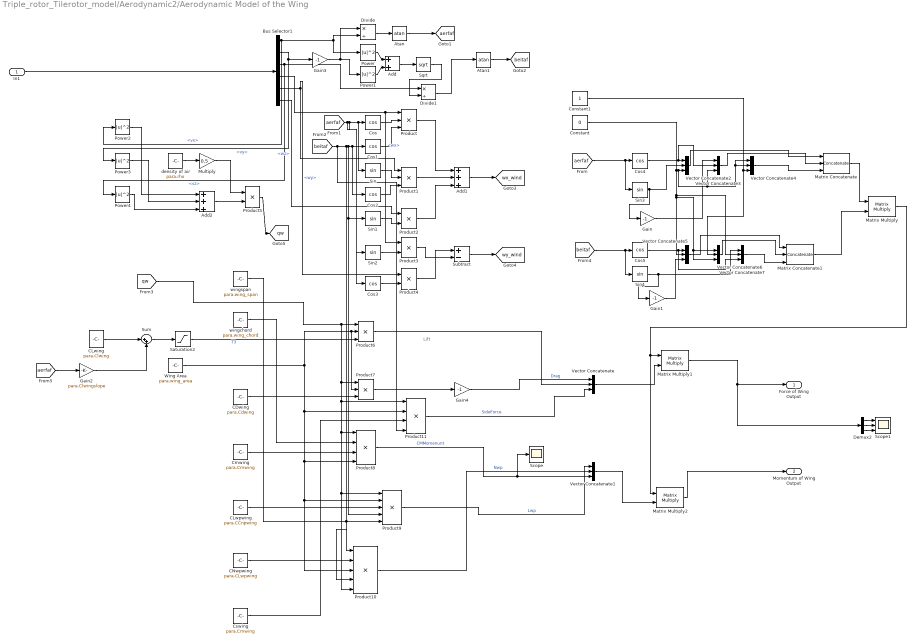
== system Triple_rotor_Tilerotor_model/Aerodynamic2/Aerodynamic Model of the Wing ==
  note: Lift
  In1 : Inport
  Add : Sum
  Add1 : Sum  Inputs=+++
  Add2 : Sum  Inputs=+++
  Atan : Trigonometry  Operator=atan
  Atan1 : Trigonometry  Operator=atan
  Bus Selector1 : BusSelector  OutputSignals=vx,vy,vz,wx,wy,wz
  CDwing : Constant  Value=para.Cdwing
  CLwing : Constant  Value=para.Clwing
  CLwpwing : Constant  Value=para.CCnpwing
  CNwpwing : Constant  Value=para.CLwpwing
  Cmwing : Constant  Value=para.Cmwing
  Constant : Constant  Value=0
  Constant1 : Constant
  Cos{,1..5} (6 alike) : Trigonometry  Operator=cos
  Cswing : Constant  Value=para.Cmwing
  Demux2 : Demux  Outputs=3
  Divide : Product  Inputs=*/
  Divide1 : Product  Inputs=*/
  Gain{,1,3..4} (4 alike) : Gain  Gain=-1
  Gain2 : Gain  Gain=para.Clwingslope
  Matrix Concatenate : Concatenate  NumInputs=3  Mode=Multidimensional array  ConcatenateDimension=2
  Matrix Concatenate1 : Concatenate  NumInputs=3  Mode=Multidimensional array  ConcatenateDimension=2
  Matrix Multiply : Product  Multiplication=Matrix(*)
  Matrix Multiply1 : Product  Multiplication=Matrix(*)
  Matrix Multiply2 : Product  Multiplication=Matrix(*)
  Multiply : Gain  Gain=0.5
  Power{,1..4} (5 alike) : Math  Operator=magnitude^2
  Product{,1,6..7} (4 alike) : Product  Inputs=3
  Product10 : Product  Inputs=5
  Product11 : Product  Inputs=4
  Product{2..5} (4 alike) : Product
  Product8 : Product  Inputs=4
  Product9 : Product  Inputs=5
  Saturation2 : Saturate  UpperLimit=1.2  LowerLimit=-1
  Scope : Scope
  Scope1 : Scope  NumInputPorts=3
  Sin{,1..4} (5 alike) : Trigonometry
  Sqrt : Sqrt
  Subtract : Sum  Inputs=+-
  Sum : Sum  Inputs=|++
  Vector Concatenate{,1..7} (8 alike) : Concatenate  NumInputs=3
  Wing Area : Constant  Value=para.wing_area
  density of air : Constant  Value=para.rho
  wingchord : Constant  Value=para.wing_chord
  wingspan : Constant  Value=para.wing_span
  Force of Wing Output : Outport
  Momentum of Wing Output : Outport  Port=2
  tag scope: aerfaf=global, beitaf=global, qw=global, wx_wind=global, wy_wind=global
  wires:
  [qw] -> Product11/1, Product10/5, Product9/1, Product8/1, Product7/1, Product6/1
  Cos/1 -> Product/2
  Product/1 -> Add1/1
  Product4/1 -> Subtract/1
  Product11/1 -> Vector Concatenate/3  "SideForce"
  Cos1/1 -> Product/3
  [aerfaf] -> Cos3/1, Sin2/1, Sin/1, Cos/1
  Bus Selector1/4 -> Product/1, Product3/1  "<wx>"
  Cos3/1 -> Product4/2
  Divide/1 -> Atan/1
  Add/1 -> Sqrt/1
  Add2/1 -> Product5/2
  Bus Selector1/3 -> Power4/1, Divide1/1  "<vz>"
  density of air/1 -> Multiply/1
  Bus Selector1/5 -> Product4/1, Product1/1  "<wy>"
  CNwpwing/1 -> Product10/2
  [beitaf] -> Product11/4, Product10/1, Sin1/1, Product9/4, Cos2/1, Cos1/1
  wingchord/1 -> Product8/2
  Power1/1 -> Add/2
  Product9/1 -> Vector Concatenate1/1  "Lwp"
  Subtract/1 -> [wy_wind]
  Cswing/1 -> Product11/3
  Power/1 -> Add/1
  Cos2/1 -> Product1/3
  Bus Selector1/6 -> Product2/1  "<wz>"
  In1/1 -> Bus Selector1/1
  Atan1/1 -> [beitaf]
  Sin/1 -> Product1/2
  Cmwing/1 -> Product8/3
  Power3/1 -> Add2/2
  Product6/1 -> Vector Concatenate/2
  Sqrt/1 -> Divide1/2
  Bus Selector1/2 -> Power3/1, Gain3/1  "<vy>"
  Sin2/1 -> Product3/2
  Multiply/1 -> Product5/1
  Product7/1 -> Gain4/1
  Product8/1 -> Scope/1, Vector Concatenate1/3  "CMMomenunt"
  CLwpwing/1 -> Product9/3
  wingspan/1 -> Product10/4, Product9/5
  Wing Area/1 -> Product7/2, Product6/2, Product10/3, Product9/2, Product8/4, Product11/2
  Divide1/1 -> Atan1/1
  Product10/1 -> Vector Concatenate1/2  "Nwp"
  Product5/1 -> [qw]
  Bus Selector1/1 -> Power2/1, Power/1, Divide/2  "<vx>"
  Sum/1 -> Saturation2/1
  Power4/1 -> Add2/3
  CDwing/1 -> Product7/3
  Add1/1 -> [wx_wind]
  Atan/1 -> [aerfaf]
  Power2/1 -> Add2/1
  Sin1/1 -> Product2/2
  Product3/1 -> Subtract/2
  Product2/1 -> Add1/3
  Product1/1 -> Add1/2
  Vector Concatenate/1 -> Matrix Multiply1/2
  [aerfaf] -> Sin3/1, Cos4/1
  Cos4/1 -> Vector Concatenate3/2, Vector Concatenate2/1
  Sin3/1 -> Gain/1, Vector Concatenate2/2
  Constant/1 -> Vector Concatenate6/3, Vector Concatenate6/1, Vector Concatenate5/2, Vector Concatenate7/2, Vector Concatenate4/2, Vector Concatenate4/1, Vector Concatenate3/3, Vector Concatenate2/3
  Gain/1 -> Vector Concatenate3/1
  [beitaf] -> Sin4/1, Cos5/1
  Constant1/1 -> Vector Concatenate6/2, Vector Concatenate4/3
  Vector Concatenate2/1 -> Matrix Concatenate/1
  Vector Concatenate3/1 -> Matrix Concatenate/2
  Vector Concatenate4/1 -> Matrix Concatenate/3
  Vector Concatenate7/1 -> Matrix Concatenate1/3
  Cos5/1 -> Vector Concatenate7/3, Vector Concatenate5/1
  Sin4/1 -> Vector Concatenate7/1, Gain1/1
  Gain1/1 -> Vector Concatenate5/3
  Vector Concatenate5/1 -> Matrix Concatenate1/1
  Vector Concatenate6/1 -> Matrix Concatenate1/2
  Matrix Concatenate/1 -> Matrix Multiply/1
  Matrix Concatenate1/1 -> Matrix Multiply/2
  Matrix Multiply/1 -> Matrix Multiply2/1, Matrix Multiply1/1
  Vector Concatenate1/1 -> Matrix Multiply2/2
  [aerfaf] -> Gain2/1
  CLwing/1 -> Sum/1
  Gain2/1 -> Sum/2
  Gain3/1 -> Power1/1, Divide/1
  Saturation2/1 -> Product6/3  "T3"
  Gain4/1 -> Vector Concatenate/1  "Drag"
  Demux2/1 -> Scope1/1
  Demux2/2 -> Scope1/2
  Matrix Multiply1/1 -> Demux2/1, Force of Wing Output/1
  Demux2/3 -> Scope1/3
  Matrix Multiply2/1 -> Momentum of Wing Output/1

== system Triple_rotor_Tilerotor_model/Forcemix/rotor_forcemix ==
  Fl : Inport
  Ml : Inport  Port=2
  Fr : Inport  Port=3
  Mr : Inport  Port=4
  Fb : Inport  Port=5
  Mb : Inport  Port=6
  AF : Inport  Port=7
  AM : Inport  Port=8
  Bus Creator3 : BusCreator  Inputs=2
  Bus Creator4 : BusCreator  Inputs=2
  Bus Creator5 : BusCreator  Inputs=2
  Demux{1..4} (4 alike) : Demux  Outputs=3
  Gain : Gain  Gain=-1
  Gain1 : Gain  Gain=-1
  Gain2 : Gain  Gain=-1
  Scope1 : Scope  NumInputPorts=3
  Scope2 : Scope  NumInputPorts=3
  Scope3 : Scope  NumInputPorts=3
  Sum : Sum  Inputs=+++
  Sum1 : Sum  Inputs=+++
  Sum2 : Sum
  Sum3 : Sum
  Sum4 : Sum  Inputs=|++|
  Sum5 : Sum  Inputs=|++|
  Sum6 : Sum  Inputs=|++|
  Out1 : Outport
  Out2 : Outport  Port=2
  tag scope: AM=global, Mrotor=global
  wires:
  Mb/1 -> Sum1/3
  Sum/1 -> Sum2/1
  Fb/1 -> Sum/3  "Fb"
  Sum3/1 -> Out2/1
  Fl/1 -> Sum/1  "Fl"
  Fr/1 -> Sum/2  "Fr"
  Ml/1 -> Sum1/1
  Mr/1 -> Sum1/2
  AF/1 -> Sum2/2, Demux4/1
  AM/1 -> [AM], Demux3/1, Sum3/2
  Sum2/1 -> Out1/1
  Sum5/1 -> Scope1/2  "y"
  Sum6/1 -> Scope1/3  "z"
  Sum4/1 -> Scope1/1  "x"
  Demux1/1 -> Sum4/1
  Demux1/2 -> Sum5/1
  Bus Creator5/1 -> Scope3/3  "z"
  Demux2/1 -> Bus Creator3/1
  Bus Creator4/1 -> Scope3/2  "y"
  Demux3/3 -> Sum6/2, Gain2/1
  Demux2/3 -> Bus Creator5/1
  Demux2/2 -> Bus Creator4/1
  Bus Creator3/1 -> Scope3/1  "x"
  Demux3/2 -> Gain1/1, Sum5/2
  Demux3/1 -> Gain/1, Sum4/2
  Demux1/3 -> Sum6/1
  Sum1/1 -> [Mrotor], Demux2/1, Demux1/1, Sum3/1
  Gain/1 -> Bus Creator3/2
  Gain2/1 -> Bus Creator5/2
  Gain1/1 -> Bus Creator4/2
  Demux4/1 -> Scope2/1
  Demux4/2 -> Scope2/2
  Demux4/3 -> Scope2/3

== system Triple_rotor_Tilerotor_model/Rotors_dynamic/Hw_back ==
  In1 : Inport
  Constant12 : Constant  Value=para.R
  Constant13 : Constant  Value=para.R
  Constant14 : Constant  Value=para.R
  Constant15 : Constant  Value=para.rho
  Constant16 : Constant  Value=1/2
  Constant17 : Constant  Value=para.CH
  Product6 : Product  Inputs=5
  Product7 : Product
  Product8 : Product
  Product9 : Product
  Hw_back : Outport
  wires:
  Constant16/1 -> Product6/5
  Constant17/1 -> Product6/4
  Constant14/1 -> Product9/2
  Product7/1 -> Product8/2, Product8/1
  Product9/1 -> Product6/2
  Constant15/1 -> Product6/3
  Product8/1 -> Product6/1
  Constant12/1 -> Product7/2
  In1/1 -> Product7/1
  Constant13/1 -> Product9/1
  Product6/1 -> Hw_back/1

== system Triple_rotor_Tilerotor_model/Rotors_dynamic/Hw_l ==
  In1 : Inport
  Constant12 : Constant  Value=para.R
  Constant13 : Constant  Value=para.R
  Constant14 : Constant  Value=para.R
  Constant15 : Constant  Value=para.rho
  Constant16 : Constant  Value=1/2
  Constant17 : Constant  Value=para.CH
  Product6 : Product  Inputs=5
  Product7 : Product
  Product8 : Product
  Product9 : Product
  Hw_l : Outport
  wires:
  Constant16/1 -> Product6/5
  Constant17/1 -> Product6/4
  Constant14/1 -> Product9/2
  Product7/1 -> Product8/2, Product8/1
  Product9/1 -> Product6/2
  Constant15/1 -> Product6/3
  Product8/1 -> Product6/1
  Constant12/1 -> Product7/2
  In1/1 -> Product7/1
  Constant13/1 -> Product9/1
  Product6/1 -> Hw_l/1

== system Triple_rotor_Tilerotor_model/Rotors_dynamic/Hw_r ==
  In1 : Inport
  Constant12 : Constant  Value=para.R
  Constant13 : Constant  Value=para.R
  Constant14 : Constant  Value=para.R
  Constant15 : Constant  Value=para.rho
  Constant16 : Constant  Value=1/2
  Constant17 : Constant  Value=para.CH
  Product6 : Product  Inputs=5
  Product7 : Product
  Product8 : Product
  Product9 : Product
  Hw_r : Outport
  wires:
  Constant16/1 -> Product6/5
  Constant17/1 -> Product6/4
  Constant14/1 -> Product9/2
  Product7/1 -> Product8/2, Product8/1
  Product9/1 -> Product6/2
  Constant15/1 -> Product6/3
  Product8/1 -> Product6/1
  Constant12/1 -> Product7/2
  In1/1 -> Product7/1
  Constant13/1 -> Product9/1
  Product6/1 -> Hw_r/1

== system Triple_rotor_Tilerotor_model/Rotors_dynamic/Subsystem1 ==
  Hw_r : Inport
  Sw_r : Inport  Port=2
  Add : Sum
  Add1 : Sum
  Gain : Gain  Gain=-1
  Product{,1..3} (4 alike) : Product
  Trigonometric Function1 : Trigonometry
  Trigonometric Function2 : Trigonometry  Operator=cos
  Hh_r : Outport
  Sh_r : Outport  Port=2
  wires:
  Hw_r/1 -> Product2/1, Product/1
  [beta_rr] -> Trigonometric Function2/1, Trigonometric Function1/1
  Trigonometric Function2/1 -> Product3/2, Product/2
  Product/1 -> Add/1
  Product1/1 -> Add/2
  Sw_r/1 -> Product3/1, Product1/2
  Trigonometric Function1/1 -> Product2/2, Product1/1
  Product2/1 -> Gain/1
  Product3/1 -> Add1/2
  Add/1 -> Hh_r/1
  Add1/1 -> Sh_r/1
  Gain/1 -> Add1/1

== system Triple_rotor_Tilerotor_model/Rotors_dynamic/Subsystem2 ==
  Hw_l : Inport
  Sw_l : Inport  Port=2
  Add : Sum
  Add1 : Sum
  Gain1 : Gain  Gain=-1
  Product{,1..3} (4 alike) : Product
  Trigonometric Function1 : Trigonometry
  Trigonometric Function2 : Trigonometry  Operator=cos
  Hh_l : Outport
  Sh_l : Outport  Port=2
  wires:
  Hw_l/1 -> Product2/1, Product/1
  [beta_lr] -> Trigonometric Function2/1, Trigonometric Function1/1
  Trigonometric Function2/1 -> Product3/2, Product/2
  Product/1 -> Add/1
  Product1/1 -> Gain1/1
  Sw_l/1 -> Product3/1, Product1/2
  Trigonometric Function1/1 -> Product2/2, Product1/1
  Product3/1 -> Add1/2
  Add/1 -> Hh_l/1
  Add1/1 -> Sh_l/1
  Product2/1 -> Add1/1
  Gain1/1 -> Add/2

== system Triple_rotor_Tilerotor_model/Rotors_dynamic/Subsystem3 ==
  Hw_back : Inport
  Sw_back : Inport  Port=2
  Add : Sum
  Add1 : Sum
  Gain : Gain  Gain=-1
  Product{,1..3} (4 alike) : Product
  Trigonometric Function1 : Trigonometry
  Trigonometric Function2 : Trigonometry  Operator=cos
  Hh_back : Outport
  Sh_back : Outport  Port=2
  wires:
  Hw_back/1 -> Product2/1, Product/1
  [beta_back] -> Trigonometric Function2/1, Trigonometric Function1/1
  Trigonometric Function2/1 -> Product3/2, Product/2
  Product/1 -> Add/1
  Product1/1 -> Add/2
  Sw_back/1 -> Product3/1, Product1/2
  Trigonometric Function1/1 -> Product2/2, Product1/1
  Product2/1 -> Gain/1
  Product3/1 -> Add1/2
  Add/1 -> Hh_back/1
  Add1/1 -> Sh_back/1
  Gain/1 -> Add1/1

== system Triple_rotor_Tilerotor_model/Rotors_dynamic/Sw_back ==
  In1 : Inport
  Constant12 : Constant  Value=para.R
  Constant13 : Constant  Value=para.R
  Constant14 : Constant  Value=para.R
  Constant15 : Constant  Value=para.rho
  Constant16 : Constant  Value=1/2
  Constant17 : Constant  Value=para.CS
  Product6 : Product  Inputs=5
  Product7 : Product
  Product8 : Product
  Product9 : Product
  Sw_back : Outport
  wires:
  Constant16/1 -> Product6/5
  Constant17/1 -> Product6/4
  Constant14/1 -> Product9/2
  Product7/1 -> Product8/2, Product8/1
  Product9/1 -> Product6/2
  Constant15/1 -> Product6/3
  Product8/1 -> Product6/1
  Constant12/1 -> Product7/2
  In1/1 -> Product7/1
  Constant13/1 -> Product9/1
  Product6/1 -> Sw_back/1

== system Triple_rotor_Tilerotor_model/Rotors_dynamic/Sw_l ==
  In1 : Inport
  Constant12 : Constant  Value=para.R
  Constant13 : Constant  Value=para.R
  Constant14 : Constant  Value=para.R
  Constant15 : Constant  Value=para.rho
  Constant16 : Constant  Value=1/2
  Constant17 : Constant  Value=para.CS
  Product6 : Product  Inputs=5
  Product7 : Product
  Product8 : Product
  Product9 : Product
  Sw_l : Outport
  wires:
  Constant16/1 -> Product6/5
  Constant17/1 -> Product6/4
  Constant14/1 -> Product9/2
  Product7/1 -> Product8/2, Product8/1
  Product9/1 -> Product6/2
  Constant15/1 -> Product6/3
  Product8/1 -> Product6/1
  Constant12/1 -> Product7/2
  In1/1 -> Product7/1
  Constant13/1 -> Product9/1
  Product6/1 -> Sw_l/1

== system Triple_rotor_Tilerotor_model/Rotors_dynamic/Sw_r ==
  In1 : Inport
  Constant12 : Constant  Value=para.R
  Constant13 : Constant  Value=para.R
  Constant14 : Constant  Value=para.R
  Constant15 : Constant  Value=para.rho
  Constant16 : Constant  Value=1/2
  Constant17 : Constant  Value=para.CS
  Product6 : Product  Inputs=5
  Product7 : Product
  Product8 : Product
  Product9 : Product
  Sw_r : Outport
  wires:
  Constant16/1 -> Product6/5
  Constant17/1 -> Product6/4
  Constant14/1 -> Product9/2
  Product7/1 -> Product8/2, Product8/1
  Product9/1 -> Product6/2
  Constant15/1 -> Product6/3
  Product8/1 -> Product6/1
  Constant12/1 -> Product7/2
  In1/1 -> Product7/1
  Constant13/1 -> Product9/1
  Product6/1 -> Sw_r/1

== system Triple_rotor_Tilerotor_model/Rotors_dynamic/Tw_back ==
  In1 : Inport
  Constant12 : Constant  Value=para.R
  Constant13 : Constant  Value=para.R
  Constant14 : Constant  Value=para.R
  Constant15 : Constant  Value=para.rho
  Constant16 : Constant  Value=1/2
  Constant17 : Constant  Value=para.CT
  Product6 : Product  Inputs=5
  Product7 : Product
  Product8 : Product  Inputs=3
  Product9 : Product
  Sign : Signum
  Tw_back : Outport
  wires:
  Constant16/1 -> Product6/5
  Constant17/1 -> Product6/4
  Constant14/1 -> Product9/2
  Product7/1 -> Product8/2, Product8/3
  Product9/1 -> Product6/2
  Constant15/1 -> Product6/3
  Product8/1 -> Product6/1
  Constant12/1 -> Product7/2
  In1/1 -> Sign/1, Product7/1
  Constant13/1 -> Product9/1
  Product6/1 -> Tw_back/1
  Sign/1 -> Product8/1

== system Triple_rotor_Tilerotor_model/Rotors_dynamic/Tw_l ==
  In1 : Inport
  Constant12 : Constant  Value=para.R
  Constant13 : Constant  Value=para.R
  Constant14 : Constant  Value=para.R
  Constant15 : Constant  Value=para.rho
  Constant16 : Constant  Value=1/2
  Constant17 : Constant  Value=para.CT
  Product6 : Product  Inputs=5
  Product7 : Product
  Product8 : Product
  Product9 : Product
  Tw_l : Outport
  wires:
  Constant16/1 -> Product6/5
  Constant17/1 -> Product6/4
  Constant14/1 -> Product9/2
  Product7/1 -> Product8/2, Product8/1
  Product9/1 -> Product6/2
  Constant15/1 -> Product6/3
  Product8/1 -> Product6/1
  Constant12/1 -> Product7/2
  In1/1 -> Product7/1
  Constant13/1 -> Product9/1
  Product6/1 -> Tw_l/1

== system Triple_rotor_Tilerotor_model/Rotors_dynamic/Tw_r ==
  In1 : Inport
  Constant12 : Constant  Value=para.R
  Constant13 : Constant  Value=para.R
  Constant14 : Constant  Value=para.R
  Constant15 : Constant  Value=para.rho
  Constant16 : Constant  Value=1/2
  Constant17 : Constant  Value=para.CT
  Product6 : Product  Inputs=5
  Product7 : Product
  Product8 : Product
  Product9 : Product
  Tw_r : Outport
  wires:
  Constant16/1 -> Product6/5
  Constant17/1 -> Product6/4
  Constant14/1 -> Product9/2
  Product7/1 -> Product8/2, Product8/1
  Product9/1 -> Product6/2
  Constant15/1 -> Product6/3
  Product8/1 -> Product6/1
  Constant12/1 -> Product7/2
  In1/1 -> Product7/1
  Constant13/1 -> Product9/1
  Product6/1 -> Tw_r/1

== system Triple_rotor_Tilerotor_model/Subsystem/Eular_angle_calculation ==
  Bus Creator : BusCreator  Inputs=3
  Bus Selector3 : BusSelector  OutputSignals=gamma,theta,wx,wy,wz
  Product{1..6} (6 alike) : Product
  Sum1 : Sum  Inputs=|++
  Sum2 : Sum  Inputs=+-|
  Sum3 : Sum  Inputs=-+|
  cos : MATLABFcn  MATLABFcn=cos(u)
  sec : MATLABFcn  MATLABFcn=1/cos(u)
  sin : MATLABFcn  MATLABFcn=sin(u)
  tan : MATLABFcn  MATLABFcn=tan(u)
  dEular_angle : Outport
  wires:
  Bus Selector3/2 -> tan/1, sec/1  "<theta>"
  Product2/1 -> Sum2/2
  Sum3/1 -> Bus Creator/1  "dgamma"
  sin/1 -> Product2/1, Product6/1
  Bus Selector3/1 -> sin/1, cos/1  "<gamma>"
  Sum2/1 -> Product4/1, Product3/1
  tan/1 -> Product3/2
  Product1/1 -> Sum2/1
  Bus Selector3/3 -> Sum3/2  "<wx>"
  Bus Selector3/5 -> Product5/2, Product2/2  "<wz>"
  Bus Selector3/4 -> Product1/2, Product6/2  "<wy>"
  [state] -> Bus Selector3/1
  Product3/1 -> Sum3/1
  sec/1 -> Product4/2
  Product4/1 -> Bus Creator/2  "dpsi"
  cos/1 -> Product5/1, Product1/1
  Product6/1 -> Sum1/1
  Product5/1 -> Sum1/2
  Sum1/1 -> Bus Creator/3  "dtheta"
  Bus Creator/1 -> dEular_angle/1
